simulink model "ejemplo1"  (R2019a)
settings: Solver=VariableStepAuto  StartTime=0.0  StopTime=20  RelTol=1e-3
settings Model: Creator=cmparedes  LastModifiedBy=cmparedes

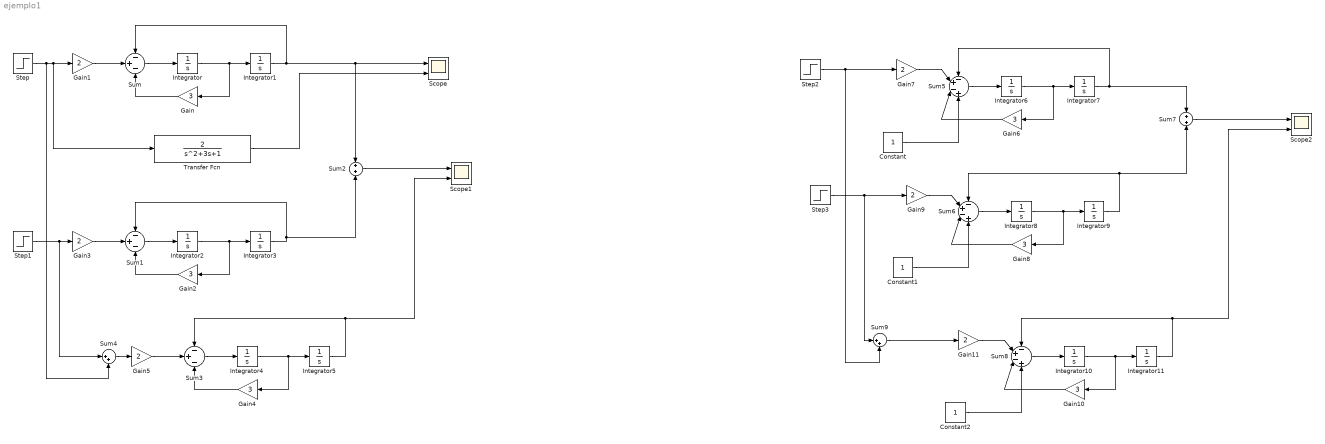
== system ejemplo1 ==
  Constant : Constant
  Constant1 : Constant
  Constant2 : Constant
  Gain{,2,4,6,8,10} (6 alike) : Gain  Gain=3
  Gain{1,3,5,7,9,11} (6 alike) : Gain  Gain=2
  Integrator{,1..11} (12 alike) : Integrator
  Scope : Scope  NumInputPorts=2
  Scope1 : Scope  NumInputPorts=2
  Scope2 : Scope  NumInputPorts=2
  Step : Step  Time=0  After=45  SampleTime=0
  Step1 : Step  Time=0  After=-10  SampleTime=0
  Step2 : Step  Time=0  After=2  SampleTime=0
  Step3 : Step  Time=0  After=-7.2  SampleTime=0
  Sum : Sum  Inputs=-+-
  Sum1 : Sum  Inputs=-+-
  Sum2 : Sum
  Sum3 : Sum  Inputs=-+-
  Sum4 : Sum  Inputs=|++
  Sum5 : Sum  Inputs=-+-+
  Sum6 : Sum  Inputs=-+-+
  Sum7 : Sum
  Sum8 : Sum  Inputs=-+-+
  Sum9 : Sum  Inputs=|++
  Transfer Fcn : TransferFcn  Numerator=2  Denominator=[1 3 1]
  wires:
  Gain1/1 -> Sum/2
  Sum/1 -> Integrator/1
  Integrator1/1 -> Sum/1, Sum2/1, Scope/1
  Gain/1 -> Sum/3
  Integrator/1 -> Gain/1, Integrator1/1
  Step/1 -> Sum4/2, Transfer Fcn/1, Gain1/1
  Transfer Fcn/1 -> Scope/2
  Step1/1 -> Sum4/1, Gain3/1
  Sum1/1 -> Integrator2/1
  Gain2/1 -> Sum1/3
  Integrator3/1 -> Sum2/2, Sum1/1
  Integrator2/1 -> Gain2/1, Integrator3/1
  Gain3/1 -> Sum1/2
  Sum2/1 -> Scope1/1
  Sum4/1 -> Gain5/1
  Gain4/1 -> Sum3/3
  Integrator4/1 -> Gain4/1, Integrator5/1
  Gain5/1 -> Sum3/2
  Sum3/1 -> Integrator4/1
  Integrator5/1 -> Scope1/2, Sum3/1
  Step2/1 -> Sum9/2, Gain7/1
  Gain6/1 -> Sum5/3
  Integrator6/1 -> Gain6/1, Integrator7/1
  Gain7/1 -> Sum5/2
  Sum5/1 -> Integrator6/1
  Integrator7/1 -> Sum7/1, Sum5/1
  Constant/1 -> Sum5/4
  Sum6/1 -> Integrator8/1
  Constant1/1 -> Sum6/4
  Integrator8/1 -> Gain8/1, Integrator9/1
  Gain9/1 -> Sum6/2
  Integrator9/1 -> Sum7/2, Sum6/1
  Step3/1 -> Sum9/1, Gain9/1
  Gain8/1 -> Sum6/3
  Sum7/1 -> Scope2/1
  Gain10/1 -> Sum8/3
  Integrator11/1 -> Scope2/2, Sum8/1
  Constant2/1 -> Sum8/4
  Sum9/1 -> Gain11/1
  Sum8/1 -> Integrator10/1
  Gain11/1 -> Sum8/2
  Integrator10/1 -> Gain10/1, Integrator11/1
